simulink model "ModelPlant_DP_v3"  (R2015a)
settings: Solver=ode3  StartTime=0.0  StopTime=Simulation_Time  FixedStep=0.01  RelTol=1e-3
values from neighbouring files (symbols this model uses):
  DesiredPath = 0    [Innput.m]    (also in Input_v3.m = 1)
  Elipscenter_radi = [6 5;0 3 ]    [Innput.m]    (also in Input_v3.m)
  eta_dot_ini = [7;0;0]    [Innput.m]    (also in Input_v3.m)
  K = [2;10]    [Input_v3.m]
  K1 = diag([1,1,4])    [Input_v3.m]
  K2 = diag([200,50,3])    [Input_v3.m]    (also in inputDPgains.m = [1 0 0; 0 1 0; 0 0 1])
  l1 = [1 0 0;0 1 0;0 0 0.05]    [Input_v3.m]    (also in inputDPgains.m = [1 0 0; 0 1 0; 0 0 0.05])
  l2 = [1 0 0;0 1 0;0 0 0.05]    [Input_v3.m]    (also in inputDPgains.m = [1 0 0; 0 1 0; 0 0 0.05])
  l3 = [1 0 0;0 1 0;0 0 0.05]    [Input_v3.m]    (also in inputDPgains.m = [1 0 0; 0 1 0; 0 0 0.05])
  L_1 = 0.1    [Input_v3.m]
  L_2 = 2    [Input_v3.m]
  L_3 = 0.01    [Input_v3.m]
  LAW = 1    [Innput.m]    (also in Input_v3.m = 0)
  lim = [1.00;-20;6.45/2;-6.45/2]    [Innput.m]    (also in Input_v3.m = [20;-20;9;-9])
  lim_2 = [1.5;-22;7;-7]    [Innput.m]    (also in Input_v3.m = [25;-25;10;-10])
  m = 14.79    [Input_v3.m]    (also in ctrl_student_init.m)
  mu = mu(1)    [Innput.m]    (also in Input_v3.m = mu(2))
  pd = [2 10;0 4]    [Input_v3.m]
  T_initialDP = T_initialDP*100    (= 0)    [Input_v3.m]
  U_ref = 0.1    [Innput.m]    (also in Input_v3.m)
(part 1 of 2)
settings Model: CovSFcnEnable=off  Creator=Erik  LastModifiedBy=MCLab
settings DebuggingCC: SolverPrmCheckMsg=warning

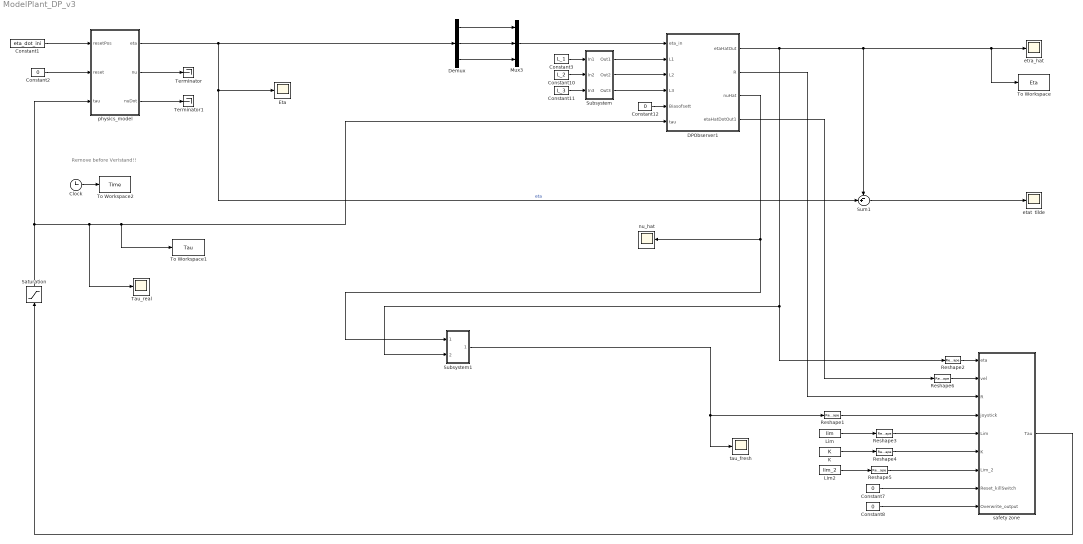
== system ModelPlant_DP_v3 ==
  note: Remove before Veristand!!
  Clock : Clock
  Constant1 : Constant  Value=eta_dot_ini
  Constant10 : Constant  Value=L_2
  Constant11 : Constant  Value=L_3
  Constant{2,7..8,12} (4 alike) : Constant  Value=0
  Constant3 : Constant  Value=L_1
  DPObserver1 : Subsystem
  Demux : Demux  Outputs=3
  Eta : Scope
      settings: TimeRange=1500  YMin=0  YMax=12  SaveName=ScopeData10
  K : Constant  Value=K
  Lim : Constant  Value=lim
  Lim2 : Constant  Value=lim_2
  Mux3 : Mux  Inputs=3
  Reshape1 : Reshape  OutputDimensionality=Customize  OutputDimensions=[3,1]
  Reshape2 : Reshape  OutputDimensionality=Customize  OutputDimensions=[3,1]
  Reshape3 : Reshape  OutputDimensionality=Customize  OutputDimensions=[4,1]
  Reshape4 : Reshape  OutputDimensionality=Customize  OutputDimensions=[2,1]
  Reshape5 : Reshape  OutputDimensionality=Customize  OutputDimensions=[4,1]
  Reshape6 : Reshape  OutputDimensionality=Customize  OutputDimensions=[3,1]
  Saturation : Saturate  UpperLimit=[1.03;2.5;0.98]  LowerLimit=-[1.03;2.5;0.98]
  Subsystem : Subsystem
  Subsystem1 : Subsystem
  Sum1 : Sum  Inputs=-+|
  Tau_real : Scope
      settings: YMin=-5e-05  YMax=0.0004  SaveName=ScopeData9
  Terminator : Terminator
  Terminator1 : Terminator
  To Workspace : ToWorkspace  VariableName=Eta  SampleTime=-1
  To Workspace1 : ToWorkspace  VariableName=Tau  SampleTime=-1
  To Workspace2 : ToWorkspace  VariableName=Time  SampleTime=-1
  etat  tilde : Scope
      settings: SaveName=ScopeData7
  etra_hat : Scope
      settings: YMin=0  YMax=25  SaveName=ScopeData5
  nu_hat : Scope
      settings: YMin=0  YMax=25  SaveName=ScopeData15
  physics_model : Subsystem
  "safety zone " : Subsystem
  tau_fresh : Scope
      settings: YMin=0  YMax=25  SaveName=ScopeData11
  wires:
  Demux/3 -> Mux3/3
  physics_model/1(eta) -> Sum1/2, Eta/1, Demux/1  "eta"
  Demux/1 -> Mux3/1
  Demux/2 -> Mux3/2
  Mux3/1 -> DPObserver1/1(eta_in)
  DPObserver1/3(nuHat) -> Subsystem1/1(nu_hat), nu_hat/1
  DPObserver1/4(etaHatDotOut1) -> Reshape6/1
  Subsystem/1(Out1) -> DPObserver1/2(L1)
  Subsystem/2(Out2) -> DPObserver1/3(L2)
  Subsystem/3(Out3) -> DPObserver1/4(L3)
  Constant7/1 -> "safety zone "/8(Reset_killSwitch)
  Constant8/1 -> "safety zone "/9(Overwrite_output)
  Lim/1 -> Reshape3/1
  K/1 -> Reshape4/1
  Lim2/1 -> Reshape5/1
  Reshape3/1 -> "safety zone "/5(Lim)
  Reshape4/1 -> "safety zone "/6(K)
  Reshape5/1 -> "safety zone "/7(Lim_2)
  Reshape1/1 -> "safety zone "/4(joystick)
  DPObserver1/2(R) -> "safety zone "/3(R)
  Reshape6/1 -> "safety zone "/2("vel ")
  Reshape2/1 -> "safety zone "/1(eta)
  Constant1/1 -> physics_model/1(resetPos)
  Constant2/1 -> physics_model/2(reset)
  physics_model/2(nu) -> Terminator/1
  physics_model/3(nuDot) -> Terminator1/1
  Constant3/1 -> Subsystem/1(In1)
  Constant11/1 -> Subsystem/3(In3)
  Constant10/1 -> Subsystem/2(In2)
  Constant12/1 -> DPObserver1/5(Biasofsett)
  "safety zone "/1(Tau) -> Saturation/1
  Saturation/1 -> physics_model/3(tau), Tau_real/1, To Workspace1/1, DPObserver1/6(tau)
  DPObserver1/1(etaHatOut) -> Reshape2/1, Subsystem1/2(Eta_hat), Sum1/1, To Workspace/1, etra_hat/1
  Sum1/1 -> etat  tilde/1
  Clock/1 -> To Workspace2/1
  Subsystem1/1(Tau) -> tau_fresh/1, Reshape1/1

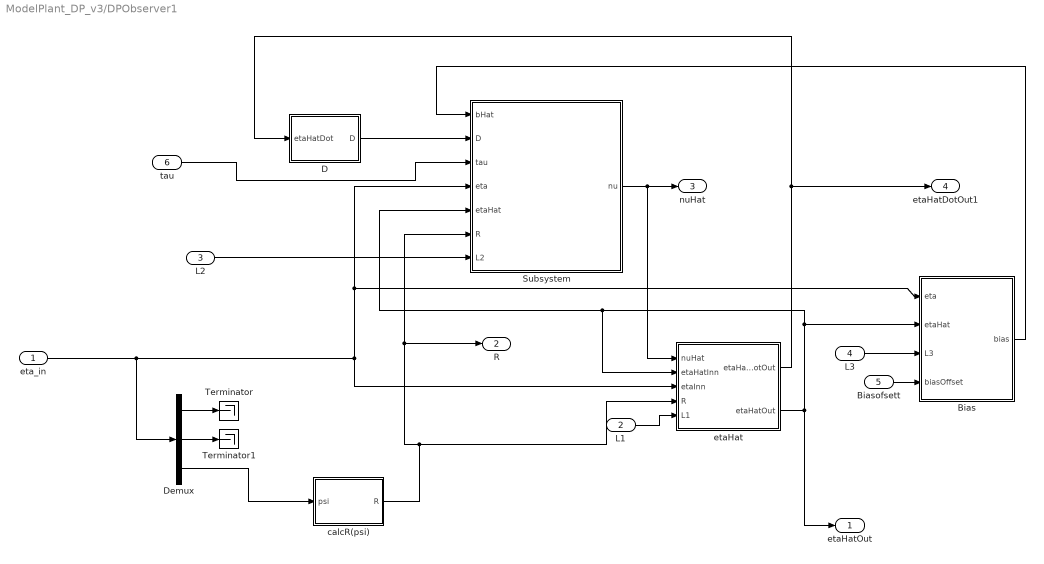
== system ModelPlant_DP_v3/DPObserver1 ==
  eta_in : Inport
  L1 : Inport  Port=2
  L2 : Inport  Port=3
  L3 : Inport  Port=4
  Biasofsett : Inport  Port=5
  tau : Inport  Port=6
  Bias : Subsystem
  D : MATLAB Function  TreatAsAtomicUnit=on
  Demux : Demux  Outputs=3
  Subsystem : Subsystem
  Terminator : Terminator
  Terminator1 : Terminator
  "calcR(psi) " : MATLAB Function  TreatAsAtomicUnit=on
  etaHat : Subsystem
  etaHatOut : Outport
  R : Outport  Port=2
  nuHat : Outport  Port=3
  etaHatDotOut1 : Outport  Port=4
  wires:
  "calcR(psi) "/1(R) -> R/1, Subsystem/6(R), etaHat/4(R)
  etaHat/2(etaHatOut) -> etaHatOut/1, Subsystem/5(etaHat), etaHat/2(etaHatInn), Bias/2(etaHat)
  tau/1 -> Subsystem/3(tau)
  etaHat/1(etaHatDotOut) -> etaHatDotOut1/1, D/1(etaHatDot)
  Subsystem/1(nu) -> nuHat/1, etaHat/1(nuHat)
  eta_in/1 -> Demux/1, etaHat/3(etaInn), Subsystem/4(eta), Bias/1(eta)
  D/1(D) -> Subsystem/2(D)
  Bias/1(bias) -> Subsystem/1(bHat)
  Demux/3 -> "calcR(psi) "/1(psi)
  L2/1 -> Subsystem/7(L2)
  L3/1 -> Bias/3(L3)
  Biasofsett/1 -> Bias/4(biasOffset)
  Demux/1 -> Terminator/1
  Demux/2 -> Terminator1/1
  L1/1 -> etaHat/5(L1)

== system ModelPlant_DP_v3/Subsystem ==
  In1 : Inport
  In2 : Inport  Port=2
  In3 : Inport  Port=3
  Constant1 : Constant  Value=l1
  Constant2 : Constant  Value=l2
  Constant3 : Constant  Value=l3
  Product : Product
  Product1 : Product
  Product2 : Product
  Out1 : Outport
  Out2 : Outport  Port=2
  Out3 : Outport  Port=3
  wires:
  Product/1 -> Out3/1
  Product2/1 -> Out2/1
  In3/1 -> Product/1
  Constant3/1 -> Product/2
  In2/1 -> Product2/1
  Constant2/1 -> Product2/2
  In1/1 -> Product1/1
  Constant1/1 -> Product1/2
  Product1/1 -> Out1/1

== system ModelPlant_DP_v3/Subsystem1 ==
  nu_hat : Inport
  Eta_hat : Inport  Port=2
  Controller1 : Subsystem
  Eta_dss : Scope
      settings: YMin=-2  YMax=10  SaveName=ScopeData14
  PathParameterization : Subsystem
  To Workspace3 : ToWorkspace  VariableName=pd_data  SampleTime=-1
  Tau : Outport
  wires:
  nu_hat/1 -> Controller1/1(nu_hat)
  Eta_hat/1 -> Controller1/8(eta_hat)
  Controller1/1("V_1s ") -> PathParameterization/1(V_1s)
  PathParameterization/3(s_dot) -> Controller1/4(s_dot)
  PathParameterization/2(U_s) -> Controller1/3(U_s)
  PathParameterization/1(eta_ds) -> Controller1/2("eta_ds ")
  PathParameterization/6(p_d_out) -> To Workspace3/1, Eta_dss/1, Controller1/7(p_d_in)
  PathParameterization/4(eta_dss) -> Controller1/5(eta_dss)
  PathParameterization/5(U_ss) -> Controller1/6(U_ss)
  Controller1/2(tau) -> Tau/1

== system ModelPlant_DP_v3/physics_model ==
  resetPos : Inport
  reset : Inport  Port=2
  tau : Inport  Port=3
  Integrator : Integrator  ExternalReset=rising  InitialCondition=[0 0 0]'
  Integrator1 : Integrator  ExternalReset=rising  InitialConditionSource=external  InitialCondition=[0 0 0]'
  Reshape1 : Reshape  OutputDimensionality=Customize  OutputDimensions=[3,1]
  Reshape3 : Reshape  OutputDimensionality=Customize  OutputDimensions=[3,1]
  kinematics : MATLAB Function  TreatAsAtomicUnit=on
  kinetics : MATLAB Function  TreatAsAtomicUnit=on
  eta : Outport
  nu : Outport  Port=2
  nuDot : Outport  Port=3
  wires:
  kinetics/1(nu_dot) -> nuDot/1, Integrator/1
  Integrator/1 -> nu/1, kinetics/2(nu), Reshape3/1
  kinematics/1(eta_dot) -> Integrator1/1
  reset/1 -> Integrator1/2, Integrator/2
  resetPos/1 -> Integrator1/3
  tau/1 -> kinetics/1(tau)
  Reshape3/1 -> kinematics/1(nu)
  Reshape1/1 -> kinematics/2(eta)
  Integrator1/1 -> Reshape1/1, eta/1

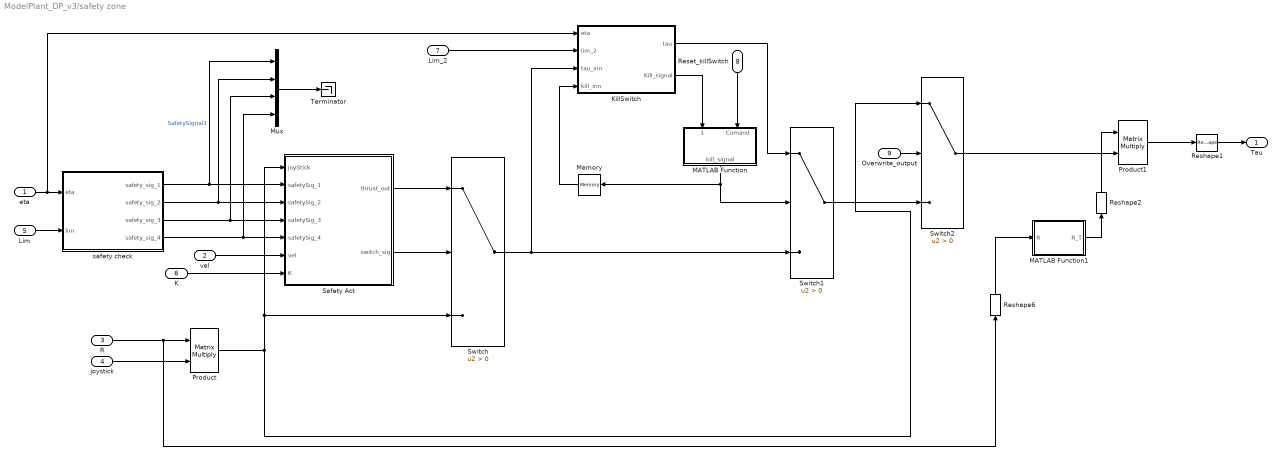
== system ModelPlant_DP_v3/safety zone  ==
  eta : Inport
  "vel " : Inport  Port=2
  R : Inport  Port=3
  joystick : Inport  Port=4
  Lim : Inport  Port=5
  K : Inport  Port=6
  Lim_2 : Inport  Port=7
  Reset_killSwitch : Inport  Port=8
  Overwrite_output : Inport  Port=9
  KillSwitch : MATLAB Function  TreatAsAtomicUnit=on
  MATLAB Function : MATLAB Function  TreatAsAtomicUnit=on
  MATLAB Function1 : MATLAB Function  TreatAsAtomicUnit=on
  Memory : Memory
  Mux : Mux
  Product : Product  Multiplication=Matrix(*)
  Product1 : Product  Multiplication=Matrix(*)
  Reshape1 : Reshape  OutputDimensionality=Customize  OutputDimensions=[3,1]
  Reshape2 : Reshape  OutputDimensionality=Customize  OutputDimensions=[3,3]
  Reshape6 : Reshape  OutputDimensionality=Customize  OutputDimensions=[3,3]
  Safety Act : MATLAB Function  TreatAsAtomicUnit=on
  Switch : Switch  Criteria=u2 > Threshold
  Switch1 : Switch  Criteria=u2 > Threshold
  Switch2 : Switch  Criteria=u2 > Threshold
  Terminator : Terminator
  safety check : MATLAB Function  TreatAsAtomicUnit=on
  Tau : Outport
  wires:
  safety check/1(safety_sig_1) -> Mux/1, Safety Act/2(safetySig_1)  "SafetySignal1"
  Safety Act/1(thrust_out) -> Switch/1
  safety check/2(safety_sig_2) -> Mux/2, Safety Act/3(safetySig_2)
  safety check/3(safety_sig_3) -> Safety Act/4(safetySig_3), Mux/3
  safety check/4(safety_sig_4) -> Safety Act/5(safetySig_4), Mux/4
  "vel "/1 -> Safety Act/6(vel)
  Mux/1 -> Terminator/1
  Lim/1 -> safety check/2(lim)
  Safety Act/2(switch_sig) -> Switch/2
  K/1 -> Safety Act/7(K)
  eta/1 -> KillSwitch/1(eta), safety check/1(eta)
  Lim_2/1 -> KillSwitch/2(lim_2)
  Memory/1 -> KillSwitch/4(kill_inn)
  Switch/1 -> KillSwitch/3(tau_inn), Switch1/3
  KillSwitch/1(tau) -> Switch1/1
  MATLAB Function/1(kill_signal) -> Memory/1, Switch1/2
  Reset_killSwitch/1 -> MATLAB Function/2(Comand)
  Overwrite_output/1 -> Switch2/2
  Switch1/1 -> Switch2/3
  KillSwitch/2(Kill_signal) -> MATLAB Function/1(kill_signalInn)
  R/1 -> Reshape6/1, Product/1
  joystick/1 -> Product/2
  Product/1 -> Safety Act/1(joyStick), Switch/3, Switch2/1
  MATLAB Function1/1(R_T) -> Reshape2/1
  Product1/1 -> Reshape1/1
  Reshape1/1 -> Tau/1
  Switch2/1 -> Product1/2
  Reshape6/1 -> MATLAB Function1/1(R)
  Reshape2/1 -> Product1/1

== system ModelPlant_DP_v3/DPObserver1/Bias ==
  eta : Inport
  etaHat : Inport  Port=2
  L3 : Inport  Port=3
  biasOffset : Inport  Port=4  PortDimensions=1
  Constant : Constant  Value=[1;1;1]
  IC1 : InitialCondition  Value=[0;0;0]
  Product : Product
  Sum : Sum  Inputs=|++
  bHat : Integrator
  bHatDot : MATLAB Function  TreatAsAtomicUnit=on
  bias : Outport
  wires:
  bHatDot/1(bHatDot) -> bHat/1
  eta/1 -> bHatDot/2(eta)
  etaHat/1 -> bHatDot/3(etaHat)
  L3/1 -> bHatDot/1(L3)
  IC1/1 -> bias/1
  Sum/1 -> IC1/1
  biasOffset/1 -> Product/1
  Product/1 -> Sum/2
  Constant/1 -> Product/2
  bHat/1 -> Sum/1

== system ModelPlant_DP_v3/DPObserver1/Subsystem ==
  bHat : Inport
  D : Inport  Port=2
  tau : Inport  Port=3
  eta : Inport  Port=4
  etaHat : Inport  Port=5
  R : Inport  Port=6
  L2 : Inport  Port=7
  IC : InitialCondition  Value=[0;0;0]
  M : MATLAB Function  TreatAsAtomicUnit=on
  nuHat : Integrator  InitialCondition=[0;0;0]
  nuHatDot : MATLAB Function  TreatAsAtomicUnit=on
  nu : Outport
  wires:
  tau/1 -> nuHatDot/6(tau)
  bHat/1 -> nuHatDot/2(bHat)
  M/1(M) -> nuHatDot/4(M)
  nuHat/1 -> nuHatDot/1(nuHat), nu/1
  etaHat/1 -> nuHatDot/9(etaHat)
  R/1 -> nuHatDot/8(R)
  eta/1 -> nuHatDot/7(eta)
  nuHatDot/1(nuHatDot) -> IC/1
  D/1 -> nuHatDot/3(D)
  L2/1 -> nuHatDot/5(L2)
  IC/1 -> nuHat/1

== system ModelPlant_DP_v3/DPObserver1/etaHat ==
  nuHat : Inport
  etaHatInn : Inport  Port=2
  etaInn : Inport  Port=3
  R : Inport  Port=4
  L1 : Inport  Port=5
  etaHat : Integrator  InitialCondition=eta_dot_ini
  etaHatDot : MATLAB Function  TreatAsAtomicUnit=on
  etaHatDotOut : Outport
  etaHatOut : Outport  Port=2
  wires:
  etaHat/1 -> etaHatOut/1
  etaHatDot/1(etaHatDot) -> etaHat/1, etaHatDotOut/1
  L1/1 -> etaHatDot/3(L1)
  R/1 -> etaHatDot/5(R)
  nuHat/1 -> etaHatDot/2(nuHat)
  etaInn/1 -> etaHatDot/4(eta)
  etaHatInn/1 -> etaHatDot/1(etaHat)

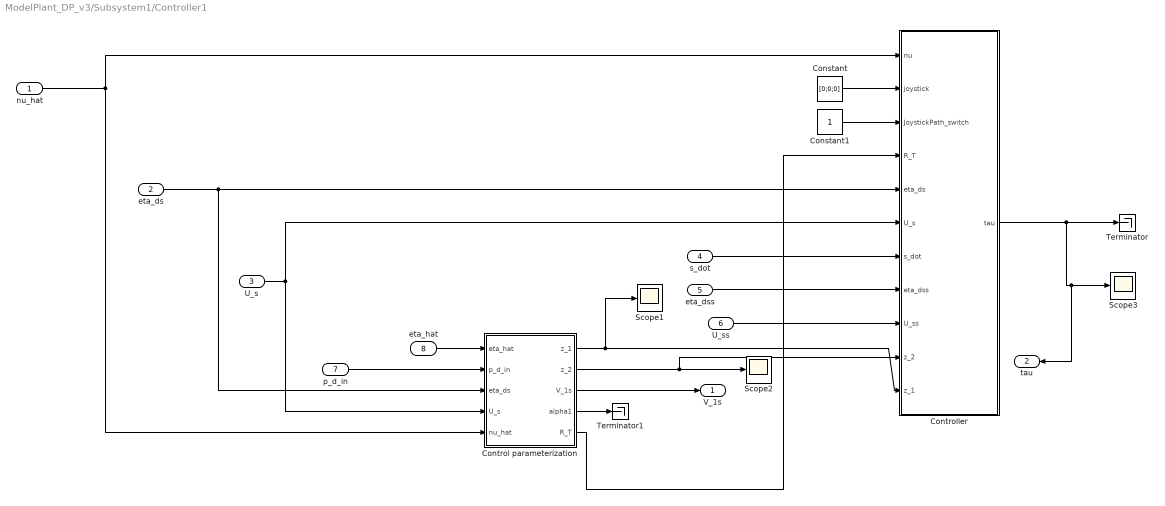
== system ModelPlant_DP_v3/Subsystem1/Controller1 ==
  nu_hat : Inport
  "eta_ds " : Inport  Port=2
  U_s : Inport  Port=3
  s_dot : Inport  Port=4
  eta_dss : Inport  Port=5
  U_ss : Inport  Port=6
  p_d_in : Inport  Port=7
  eta_hat : Inport  Port=8
  Constant : Constant  Value=[0;0;0]
  Constant1 : Constant
  Control parameterization : Subsystem
  Controller : Subsystem
  Scope1 : Scope
      settings: YMin=-6.76763  YMax=7.09799  SaveName=ScopeData8
  Scope2 : Scope
  Scope3 : Scope
      settings: YMin=-11.79233  YMax=2.58486  SaveName=ScopeData3
  Terminator : Terminator
  Terminator1 : Terminator
  "V_1s " : Outport
  tau : Outport  Port=2
  wires:
  Control parameterization/1(z_1) -> Scope1/1, Controller/11(z_1)
  Control parameterization/2(z_2) -> Scope2/1, Controller/10(z_2)
  nu_hat/1 -> Controller/1(" nu"), Control parameterization/5(nu_hat)
  Control parameterization/5("R_T ") -> Controller/4(R_T)
  Constant/1 -> Controller/2(joystick)
  Constant1/1 -> Controller/3(JoystickPath_switch)
  Controller/1(tau) -> tau/1, Scope3/1, Terminator/1
  Control parameterization/4(alpha1) -> Terminator1/1
  U_ss/1 -> Controller/9(U_ss)
  s_dot/1 -> Controller/7(s_dot)
  eta_dss/1 -> Controller/8(eta_dss)
  Control parameterization/3("V_1s ") -> "V_1s "/1
  U_s/1 -> Controller/6(U_s), Control parameterization/4(U_s)
  "eta_ds "/1 -> Control parameterization/3("eta_ds "), Controller/5(eta_ds)
  p_d_in/1 -> Control parameterization/2("p_d_in ")
  eta_hat/1 -> Control parameterization/1(eta_hat)

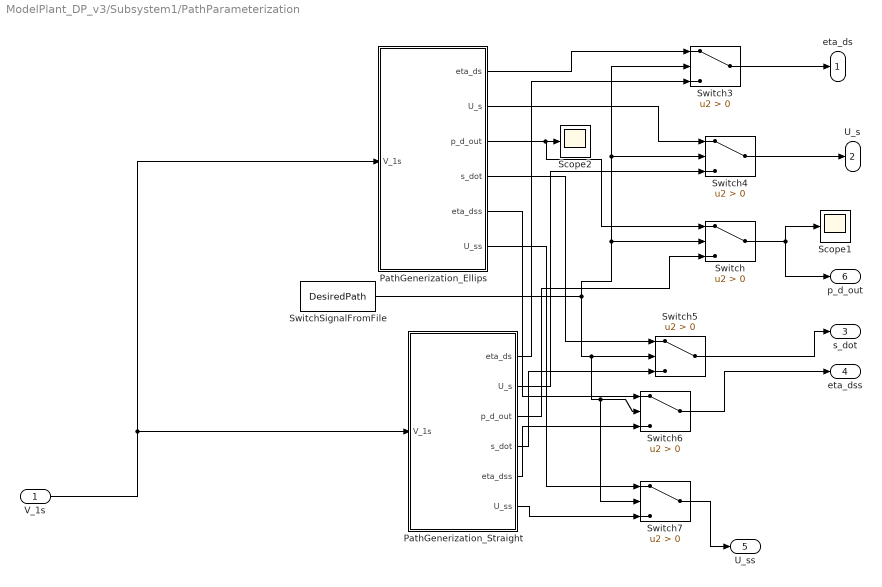
== system ModelPlant_DP_v3/Subsystem1/PathParameterization ==
  V_1s : Inport
  PathGenerization_Ellips : Subsystem
  PathGenerization_Straight : Subsystem
  Scope1 : Scope
      settings: YMin=-1.25  YMax=11.25  SaveName=ScopeData2
  Scope2 : Scope
      settings: YMin=-4.75  YMax=12.75  SaveName=ScopeData12
  Switch{,3..7} (6 alike) : Switch  Criteria=u2 > Threshold
  SwitchSignalFromFile : Constant  Value=DesiredPath
  eta_ds : Outport
  U_s : Outport  Port=2
  s_dot : Outport  Port=3
  eta_dss : Outport  Port=4
  U_ss : Outport  Port=5
  p_d_out : Outport  Port=6
  wires:
  PathGenerization_Ellips/4(s_dot) -> Switch5/1
  PathGenerization_Straight/4(s_dot) -> Switch5/3
  PathGenerization_Ellips/6(U_ss) -> Switch7/1
  PathGenerization_Straight/6(U_ss) -> Switch7/3
  PathGenerization_Straight/5("eta_dss ") -> Switch6/3
  PathGenerization_Straight/1(eta_ds) -> Switch3/3
  PathGenerization_Ellips/1(eta_ds) -> Switch3/1
  PathGenerization_Straight/2(U_s) -> Switch4/3
  PathGenerization_Straight/3(p_d_out) -> Switch/3
  PathGenerization_Ellips/2(U_s) -> Switch4/1
  PathGenerization_Ellips/3(p_d_out) -> Switch/1, Scope2/1
  SwitchSignalFromFile/1 -> Switch4/2, Switch3/2, Switch/2, Switch7/2, Switch6/2, Switch5/2
  Switch3/1 -> eta_ds/1
  Switch4/1 -> U_s/1
  Switch5/1 -> s_dot/1
  Switch6/1 -> eta_dss/1
  Switch7/1 -> U_ss/1
  V_1s/1 -> PathGenerization_Ellips/1(V_1s), PathGenerization_Straight/1(V_1s)
  Switch/1 -> p_d_out/1, Scope1/1
  PathGenerization_Ellips/5("eta_dss ") -> Switch6/1

== system ModelPlant_DP_v3/Subsystem1/Controller1/Control parameterization ==
  eta_hat : Inport
  "p_d_in " : Inport  Port=2
  "eta_ds " : Inport  Port=3
  U_s : Inport  Port=4
  nu_hat : Inport  Port=5
  "BacksteppingParameterization " : Subsystem
  z_1 : Outport
  z_2 : Outport  Port=2
  "V_1s " : Outport  Port=3
  alpha1 : Outport  Port=4
  "R_T " : Outport  Port=5
  wires:
  "eta_ds "/1 -> "BacksteppingParameterization "/3(eta_ds)
  eta_hat/1 -> "BacksteppingParameterization "/1(eta_hat)
  "p_d_in "/1 -> "BacksteppingParameterization "/2("p_d_in ")
  "BacksteppingParameterization "/1(V_1s_out) -> "V_1s "/1
  U_s/1 -> "BacksteppingParameterization "/4(U_s)
  "BacksteppingParameterization "/3(z_2) -> z_2/1
  nu_hat/1 -> "BacksteppingParameterization "/5(nu_hat)
  "BacksteppingParameterization "/2(z_1) -> z_1/1
  "BacksteppingParameterization "/4("alpha1 ") -> alpha1/1
  "BacksteppingParameterization "/5(R_T) -> "R_T "/1

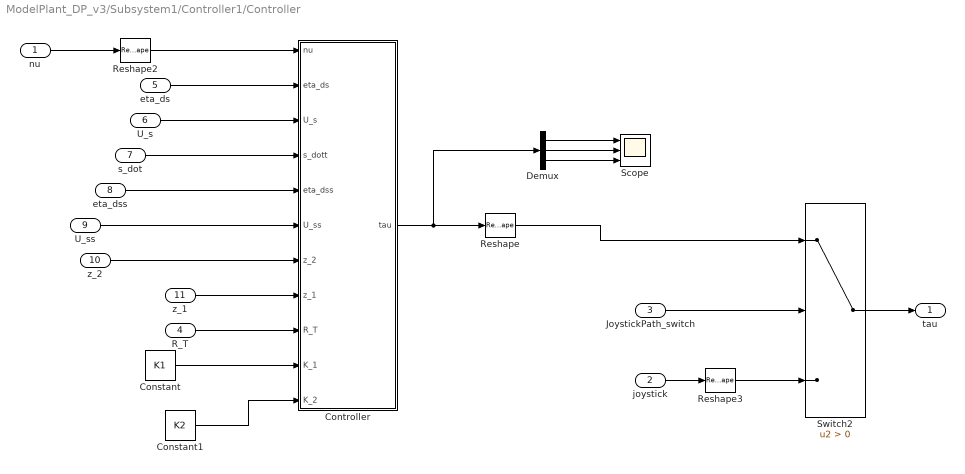
== system ModelPlant_DP_v3/Subsystem1/Controller1/Controller ==
  " nu" : Inport
  joystick : Inport  Port=2
  JoystickPath_switch : Inport  Port=3
  R_T : Inport  Port=4
  eta_ds : Inport  Port=5
  U_s : Inport  Port=6
  s_dot : Inport  Port=7
  eta_dss : Inport  Port=8
  U_ss : Inport  Port=9
  z_2 : Inport  Port=10
  z_1 : Inport  Port=11
  Constant : Constant  Value=K1
  Constant1 : Constant  Value=K2
  Controller : Subsystem
  Demux : Demux  Outputs=3
  Reshape : Reshape  OutputDimensionality=Customize  OutputDimensions=[3,1]
  Reshape2 : Reshape  OutputDimensionality=Customize  OutputDimensions=[3,1]
  Reshape3 : Reshape  OutputDimensionality=Customize  OutputDimensions=[3,1]
  Scope : Scope  NumInputPorts=3
      settings: YMin=-1.81121~-0.05182~-0.00671  YMax=5.53458~0.46636~0.06037  SaveName=ScopeData6
  Switch2 : Switch  Criteria=u2 > Threshold
  tau : Outport
  wires:
  " nu"/1 -> Reshape2/1
  Switch2/1 -> tau/1
  joystick/1 -> Reshape3/1
  JoystickPath_switch/1 -> Switch2/2
  eta_ds/1 -> Controller/2(eta_ds)
  U_s/1 -> Controller/3(U_s)
  s_dot/1 -> Controller/4(s_dott)
  eta_dss/1 -> Controller/5(eta_dss)
  U_ss/1 -> Controller/6(U_ss)
  Controller/1(tau) -> Demux/1, Reshape/1
  R_T/1 -> Controller/9(R_T)
  Constant/1 -> Controller/10(K_1)
  Constant1/1 -> Controller/11(K_2)
  Reshape/1 -> Switch2/1
  z_2/1 -> Controller/7(z_2)
  Reshape2/1 -> Controller/1(nu)
  Reshape3/1 -> Switch2/3
  z_1/1 -> Controller/8(z_1)
  Demux/1 -> Scope/1
  Demux/2 -> Scope/2
  Demux/3 -> Scope/3

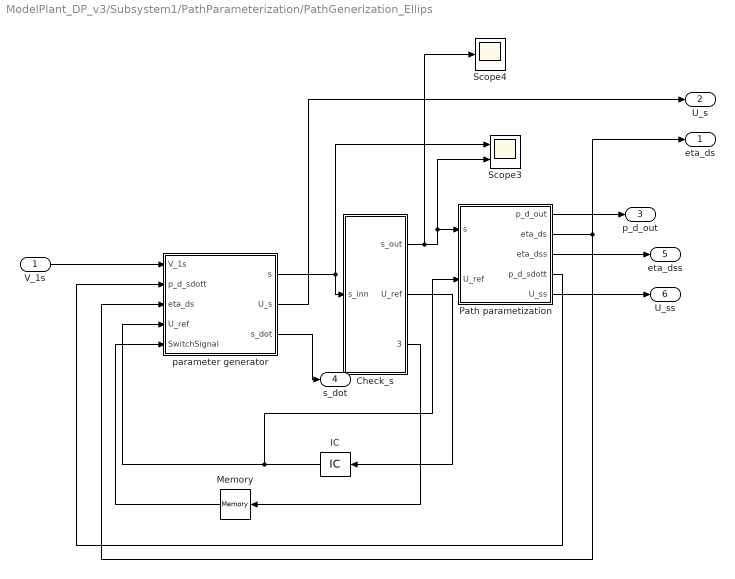
== system ModelPlant_DP_v3/Subsystem1/PathParameterization/PathGenerization_Ellips ==
  V_1s : Inport
  Check_s : Subsystem
  IC : InitialCondition  Value=0
  Memory : Memory
  "Path parametization " : Subsystem
  Scope3 : Scope  NumInputPorts=2
      settings: YMin=-0.125  YMax=1.12502  SaveName=ScopeData13
  Scope4 : Scope
  parameter generator : Subsystem
  eta_ds : Outport
  U_s : Outport  Port=2
  p_d_out : Outport  Port=3
  s_dot : Outport  Port=4
  "eta_dss " : Outport  Port=5
  U_ss : Outport  Port=6
  wires:
  "Path parametization "/1("p_d_out ") -> p_d_out/1
  parameter generator/1(s) -> Scope3/1, Check_s/1(s_inn)
  "Path parametization "/4(p_d_sdott) -> parameter generator/2(p_d_sdott)
  parameter generator/2(U_s) -> U_s/1
  "Path parametization "/2("eta_ds ") -> parameter generator/3(eta_ds), eta_ds/1
  V_1s/1 -> parameter generator/1(V_1s)
  Check_s/1(s_out) -> Scope4/1, Scope3/2, "Path parametization "/1(s)
  Check_s/2(U_ref) -> IC/1
  IC/1 -> "Path parametization "/2(U_ref), parameter generator/4(U_ref)
  Memory/1 -> parameter generator/5(SwitchSignal)
  Check_s/3(SwitchSignal) -> Memory/1
  parameter generator/3("s_dot ") -> s_dot/1
  "Path parametization "/3(eta_dss) -> "eta_dss "/1
  "Path parametization "/5(U_ss) -> U_ss/1

== system ModelPlant_DP_v3/Subsystem1/PathParameterization/PathGenerization_Straight ==
  V_1s : Inport
  IC : InitialCondition  Value=0
  Memory : Memory
  "Path parametization " : Subsystem
  Scope1 : Scope
  Scope3 : Scope
  parameter generator : Subsystem
  eta_ds : Outport
  U_s : Outport  Port=2
  p_d_out : Outport  Port=3
  s_dot : Outport  Port=4
  "eta_dss " : Outport  Port=5
  U_ss : Outport  Port=6
  wires:
  "Path parametization "/1("p_d_out ") -> p_d_out/1
  "Path parametization "/3(p_d_sdott) -> parameter generator/2(p_d_sdott)
  "Path parametization "/2("eta_ds ") -> parameter generator/3(eta_ds), eta_ds/1
  V_1s/1 -> parameter generator/1(V_1s)
  parameter generator/1(s) -> Scope3/1, "Path parametization "/1(s)
  IC/1 -> parameter generator/4(U_ref)
  Memory/1 -> parameter generator/5(SwitchSignal)
  "Path parametization "/4(SwitchSignal) -> Memory/1
  parameter generator/3("s_dot ") -> s_dot/1
  "Path parametization "/5(eta_dss) -> "eta_dss "/1
  "Path parametization "/6(U_ss) -> U_ss/1
  parameter generator/2(U_s) -> Scope1/1, U_s/1
  "Path parametization "/7(U) -> IC/1

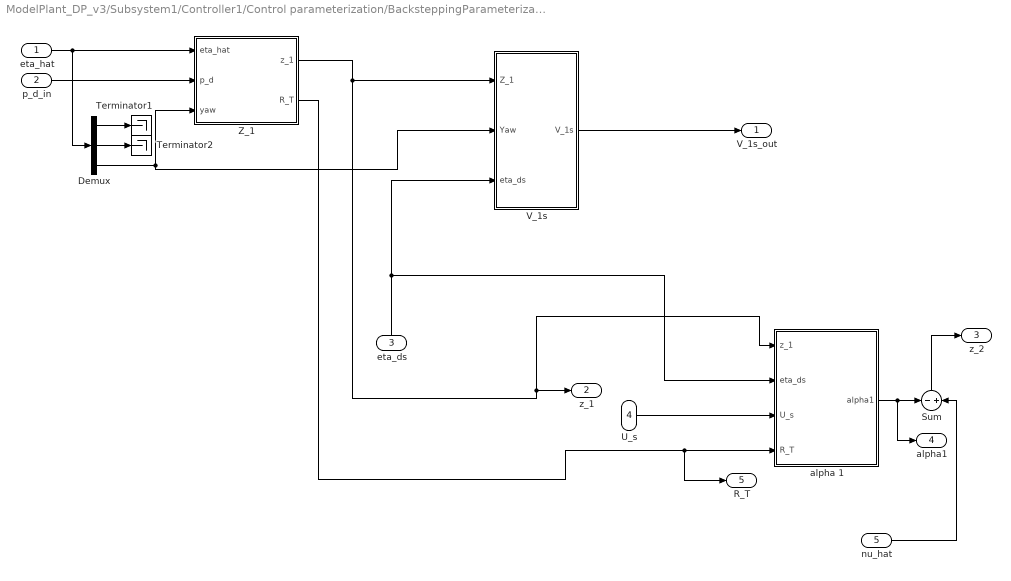
== system ModelPlant_DP_v3/Subsystem1/Controller1/Control parameterization/BacksteppingParameterization  ==
  eta_hat : Inport
  "p_d_in " : Inport  Port=2
  eta_ds : Inport  Port=3
  U_s : Inport  Port=4
  nu_hat : Inport  Port=5
  Demux : Demux  Outputs=3
  Sum : Sum  Inputs=-|+
  Terminator1 : Terminator
  Terminator2 : Terminator
  V_1s : Subsystem
  Z_1 : Subsystem
  alpha 1 : Subsystem
  V_1s_out : Outport
  z_1 : Outport  Port=2
  z_2 : Outport  Port=3
  "alpha1 " : Outport  Port=4
  R_T : Outport  Port=5
  wires:
  eta_ds/1 -> alpha 1/2(eta_ds), V_1s/3(eta_ds)
  eta_hat/1 -> Demux/1, Z_1/1(eta_hat)
  "p_d_in "/1 -> Z_1/2(p_d)
  Demux/3 -> V_1s/2(Yaw), Z_1/3("yaw ")
  V_1s/1(V_1s) -> V_1s_out/1
  alpha 1/1(alpha1) -> "alpha1 "/1, Sum/1
  U_s/1 -> alpha 1/3(U_s)
  Z_1/1(z_1) -> alpha 1/1(z_1), z_1/1, V_1s/1(Z_1)
  Z_1/2(R_T) -> R_T/1, alpha 1/4(R_T)
  nu_hat/1 -> Sum/2
  Sum/1 -> z_2/1
  Demux/1 -> Terminator1/1
  Demux/2 -> Terminator2/1

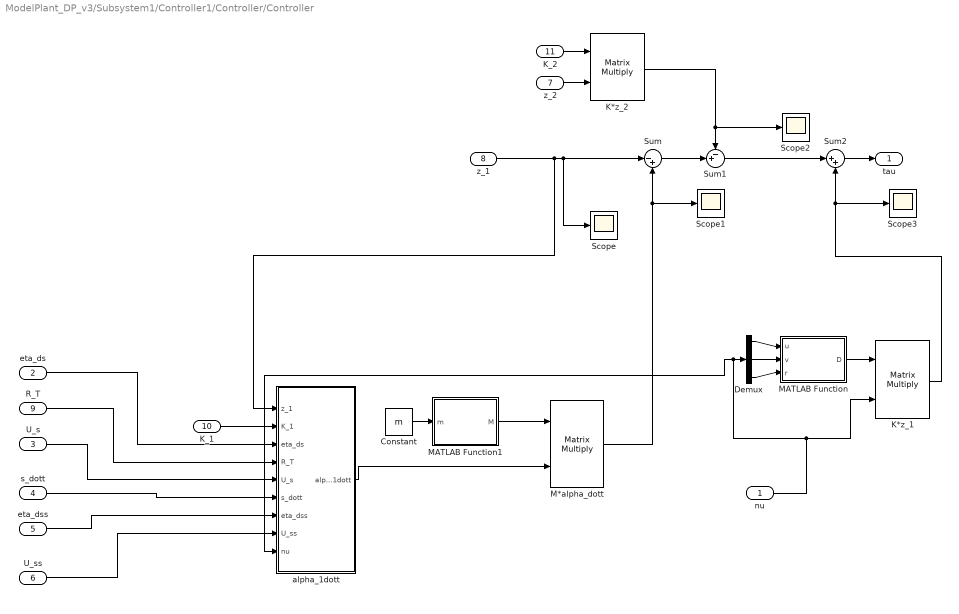
== system ModelPlant_DP_v3/Subsystem1/Controller1/Controller/Controller ==
  nu : Inport
  eta_ds : Inport  Port=2
  U_s : Inport  Port=3
  s_dott : Inport  Port=4
  eta_dss : Inport  Port=5
  U_ss : Inport  Port=6
  z_2 : Inport  Port=7
  z_1 : Inport  Port=8
  R_T : Inport  Port=9
  K_1 : Inport  Port=10
  K_2 : Inport  Port=11
  Constant : Constant  Value=m
  Demux : Demux  Outputs=3
  K*z_1 : Product  Multiplication=Matrix(*)
  K*z_2 : Product  Multiplication=Matrix(*)
  M*alpha_dott : Product  Multiplication=Matrix(*)
  MATLAB Function : MATLAB Function  TreatAsAtomicUnit=on
  MATLAB Function1 : MATLAB Function  TreatAsAtomicUnit=on
  Scope{,1..3} (4 alike) : Scope
      Scope settings: YMin=-1.86769  YMax=9.78914
      Scope1 settings: YMin=-0.31241  YMax=0.96684  SaveName=ScopeData2
      Scope2 settings: YMin=-1.22848  YMax=2.91428  SaveName=ScopeData3
      Scope3 settings: YMin=-1.62155  YMax=0.35636  SaveName=ScopeData4
  Sum : Sum  Inputs=|-+
  Sum1 : Sum  Inputs=-+|
  Sum2 : Sum  Inputs=|++
  alpha_1dott : Subsystem
  tau : Outport
  wires:
  alpha_1dott/1(alpha_1dott) -> M*alpha_dott/2
  MATLAB Function1/1(M) -> M*alpha_dott/1
  z_1/1 -> alpha_1dott/1(z_1), Scope/1, Sum/1
  Sum/1 -> Sum1/2
  Sum1/1 -> Sum2/1
  Sum2/1 -> tau/1
  z_2/1 -> K*z_2/2
  K*z_1/1 -> Sum2/2, Scope3/1
  nu/1 -> alpha_1dott/9(nu), Demux/1, K*z_1/2
  eta_ds/1 -> alpha_1dott/3(eta_ds)
  R_T/1 -> alpha_1dott/4(R_T)
  U_s/1 -> alpha_1dott/5(U_s)
  s_dott/1 -> alpha_1dott/6(s_dott)
  eta_dss/1 -> alpha_1dott/7(eta_dss)
  U_ss/1 -> alpha_1dott/8(U_ss)
  K_1/1 -> alpha_1dott/2(K_1)
  K_2/1 -> K*z_2/1
  Demux/1 -> MATLAB Function/1(u)
  Demux/2 -> MATLAB Function/2(v)
  Demux/3 -> MATLAB Function/3(r)
  MATLAB Function/1(D) -> K*z_1/1
  Constant/1 -> MATLAB Function1/1(m)
  K*z_2/1 -> Scope2/1, Sum1/1
  M*alpha_dott/1 -> Scope1/1, Sum/2

== system ModelPlant_DP_v3/Subsystem1/PathParameterization/PathGenerization_Ellips/Check_s ==
  s_inn : Inport
  CheckS&getU : MATLAB Function  TreatAsAtomicUnit=on
  Constant : Constant  Value=U_ref
  s_out : Outport
  U_ref : Outport  Port=2
  SwitchSignal : Outport  Port=3
  wires:
  CheckS&getU/1(s_out) -> s_out/1
  s_inn/1 -> CheckS&getU/1(s_inn)
  CheckS&getU/2(U) -> U_ref/1
  Constant/1 -> CheckS&getU/2(U_ref)
  CheckS&getU/3(Switch) -> SwitchSignal/1

== system ModelPlant_DP_v3/Subsystem1/PathParameterization/PathGenerization_Ellips/Path parametization  ==
  s : Inport
  U_ref : Inport  Port=2
  Elipscenter_radi : Constant  Value=Elipscenter_radi  VectorParams1D=off
  Subsystem : Subsystem
  "p_d_out " : Outport
  "eta_ds " : Outport  Port=2
  eta_dss : Outport  Port=3
  p_d_sdott : Outport  Port=4
  U_ss : Outport  Port=5
  wires:
  Elipscenter_radi/1 -> Subsystem/1(Elipscenter_radi)
  s/1 -> Subsystem/2(s)
  Subsystem/1(P_d) -> "p_d_out "/1
  Subsystem/2(Pd_s) -> p_d_sdott/1
  Subsystem/3(eta_ds) -> "eta_ds "/1
  Subsystem/4(eta_dss) -> eta_dss/1
  U_ref/1 -> Subsystem/3(U_ref)
  Subsystem/5(U_ss) -> U_ss/1

== system ModelPlant_DP_v3/Subsystem1/PathParameterization/PathGenerization_Ellips/parameter generator ==
  V_1s : Inport
  p_d_sdott : Inport  Port=2
  eta_ds : Inport  Port=3
  U_ref : Inport  Port=4
  SwitchSignal : Inport  Port=5
  Integrator : Integrator  ExternalReset=rising
  MATLAB Function1 : MATLAB Function  TreatAsAtomicUnit=on
  TASK : Constant  Value=LAW
  UpdateLaw : MATLAB Function  TreatAsAtomicUnit=on
  "mu " : Constant  Value=mu
  s : Outport
  U_s : Outport  Port=2
  "s_dot " : Outport  Port=3
  wires:
  Integrator/1 -> s/1
  p_d_sdott/1 -> UpdateLaw/1(p_d_sdot)
  UpdateLaw/1(s_dot) -> "s_dot "/1, Integrator/1
  UpdateLaw/2(U_s) -> U_s/1
  U_ref/1 -> UpdateLaw/2(U_ref)
  V_1s/1 -> UpdateLaw/3(V_1s)
  "mu "/1 -> UpdateLaw/4(mu)
  eta_ds/1 -> UpdateLaw/5(eta_ds)
  MATLAB Function1/1(SwitchSignal_Out) -> Integrator/2
  TASK/1 -> UpdateLaw/6(LAW)
  SwitchSignal/1 -> MATLAB Function1/1(SwitchSignal_In)

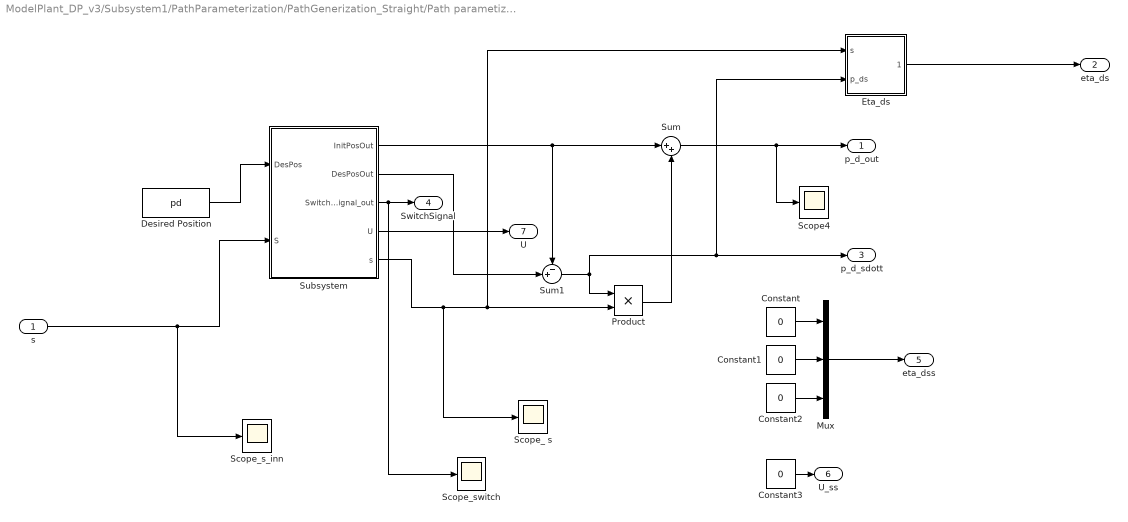
== system ModelPlant_DP_v3/Subsystem1/PathParameterization/PathGenerization_Straight/Path parametization  ==
  s : Inport
  Constant{,1..3} (4 alike) : Constant  Value=0
  Desired Position : Constant  Value=pd  VectorParams1D=off
  Eta_ds : Subsystem
  Mux : Mux  Inputs=3
  Product : Product
  Scope4 : Scope
      settings: YMin=0  YMax=12
  Scope_ s : Scope
      settings: YMin=0  YMax=1
  Scope_s_inn : Scope
      settings: TimeRange=1000  YMin=0  YMax=1.4
  Scope_switch : Scope
      settings: YMin=-0  YMax=2
  Subsystem : Subsystem
  Sum : Sum  Inputs=|++
  Sum1 : Sum  Inputs=-+|
  "p_d_out " : Outport
  "eta_ds " : Outport  Port=2
  p_d_sdott : Outport  Port=3
  SwitchSignal : Outport  Port=4
  eta_dss : Outport  Port=5
  U_ss : Outport  Port=6
  U : Outport  Port=7
  wires:
  Product/1 -> Sum/2
  Desired Position/1 -> Subsystem/1(DesPos)
  s/1 -> Scope_s_inn/1, Subsystem/2(S)
  Sum1/1 -> Product/1, Eta_ds/2(p_ds), p_d_sdott/1
  Eta_ds/1(eta_ds) -> "eta_ds "/1
  Subsystem/1(InitPosOut) -> Sum1/1, Sum/1
  Subsystem/3(SwitchSignal_out) -> Scope_switch/1, SwitchSignal/1
  Subsystem/2(DesPosOut) -> Sum1/2
  Sum/1 -> Scope4/1, "p_d_out "/1
  Mux/1 -> eta_dss/1
  Constant/1 -> Mux/1
  Constant1/1 -> Mux/2
  Constant2/1 -> Mux/3
  Constant3/1 -> U_ss/1
  Subsystem/4(U) -> U/1
  Subsystem/5(s) -> Scope_ s/1, Eta_ds/1(s), Product/2

== system ModelPlant_DP_v3/Subsystem1/PathParameterization/PathGenerization_Straight/parameter generator ==
  V_1s : Inport
  p_d_sdott : Inport  Port=2
  eta_ds : Inport  Port=3
  U_ref : Inport  Port=4
  SwitchSignal : Inport  Port=5
  Integrator : Integrator  ExternalReset=rising
  MATLAB Function1 : MATLAB Function  TreatAsAtomicUnit=on
  TASK : Constant  Value=LAW
  UpdateLaw : MATLAB Function  TreatAsAtomicUnit=on
  "mu " : Constant  Value=mu
  s : Outport
  U_s : Outport  Port=2
  "s_dot " : Outport  Port=3
  wires:
  Integrator/1 -> s/1
  p_d_sdott/1 -> UpdateLaw/1(p_d_sdot)
  UpdateLaw/1(s_dot) -> "s_dot "/1, Integrator/1
  UpdateLaw/2(U_s) -> U_s/1
  U_ref/1 -> UpdateLaw/2(U_ref)
  V_1s/1 -> UpdateLaw/3(V_1s)
  "mu "/1 -> UpdateLaw/4(mu)
  eta_ds/1 -> UpdateLaw/5(eta_ds)
  MATLAB Function1/1(SwitchSignal_Out) -> Integrator/2
  TASK/1 -> UpdateLaw/6(LAW)
  SwitchSignal/1 -> MATLAB Function1/1(SwitchSignal_In)

== system ModelPlant_DP_v3/Subsystem1/Controller1/Control parameterization/BacksteppingParameterization /V_1s ==
  Z_1 : Inport
  Yaw : Inport  Port=2
  eta_ds : Inport  Port=3
  Gain : Gain  Gain=-1
  MATLAB Function : MATLAB Function  TreatAsAtomicUnit=on
  MATLAB Function1 : MATLAB Function  TreatAsAtomicUnit=on
  Product : Product  Multiplication=Matrix(*)
  Product1 : Product  Multiplication=Matrix(*)
  Rotation Matrix : MATLAB Function  TreatAsAtomicUnit=on
  V_1s : Outport
  wires:
  Z_1/1 -> MATLAB Function/1(z_1)
  Rotation Matrix/1(R) -> MATLAB Function1/1(R)
  MATLAB Function1/1(R_T) -> Product/2
  Yaw/1 -> Rotation Matrix/1(yaw)
  MATLAB Function/1(z_1T) -> Product/1
  Product/1 -> Product1/1
  Product1/1 -> Gain/1
  eta_ds/1 -> Product1/2
  Gain/1 -> V_1s/1

== system ModelPlant_DP_v3/Subsystem1/Controller1/Control parameterization/BacksteppingParameterization /Z_1 ==
  eta_hat : Inport
  p_d : Inport  Port=2
  "yaw " : Inport  Port=3
  Mux : Mux  Inputs=2
  Product : Product  Multiplication=Matrix(*)
  R Transposed : MATLAB Function  TreatAsAtomicUnit=on
  Reshape1 : Reshape  OutputDimensionality=Customize  OutputDimensions=[3,3]
  Rotation Matrix : MATLAB Function  TreatAsAtomicUnit=on
  Sum : Sum  Inputs=|+-
  z_1 : Outport
  R_T : Outport  Port=2
  wires:
  "yaw "/1 -> Mux/2, Rotation Matrix/1(yaw)
  p_d/1 -> Mux/1
  Sum/1 -> Product/2
  Rotation Matrix/1(R) -> R Transposed/1(R)
  Product/1 -> z_1/1
  Mux/1 -> Sum/2
  R Transposed/1(R_T) -> Reshape1/1
  Reshape1/1 -> Product/1, R_T/1
  eta_hat/1 -> Sum/1

== system ModelPlant_DP_v3/Subsystem1/Controller1/Control parameterization/BacksteppingParameterization /alpha 1 ==
  z_1 : Inport
  eta_ds : Inport  Port=2
  U_s : Inport  Port=3
  R_T : Inport  Port=4
  Gain : Gain  Gain=-1
  "Kp " : Constant  Value=K1
  Product : Product  Multiplication=Matrix(*)
  Product1 : Product  Multiplication=Matrix(*)
  Product2 : Product  Multiplication=Matrix(*)
  Reshape : Reshape  OutputDimensionality=Customize  OutputDimensions=[3,1]
  Reshape1 : Reshape  OutputDimensionality=Customize
  Sum : Sum  Inputs=|++
  alpha1 : Outport
  wires:
  "Kp "/1 -> Gain/1
  Gain/1 -> Product/1
  z_1/1 -> Product/2
  Sum/1 -> alpha1/1
  Product/1 -> Sum/1
  Product1/1 -> Product2/2
  eta_ds/1 -> Reshape/1
  U_s/1 -> Reshape1/1
  Reshape/1 -> Product1/1
  Reshape1/1 -> Product1/2
  Product2/1 -> Sum/2
  R_T/1 -> Product2/1

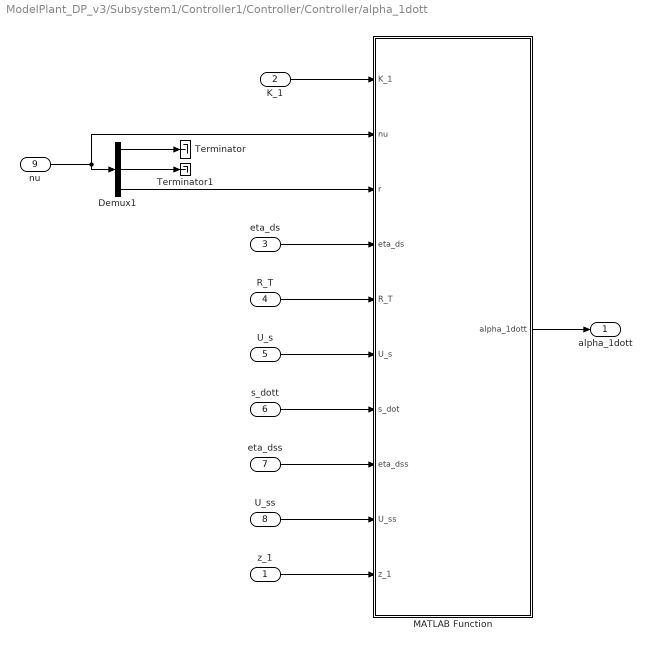
== system ModelPlant_DP_v3/Subsystem1/Controller1/Controller/Controller/alpha_1dott ==
  z_1 : Inport
  K_1 : Inport  Port=2
  eta_ds : Inport  Port=3
  R_T : Inport  Port=4
  U_s : Inport  Port=5
  s_dott : Inport  Port=6
  eta_dss : Inport  Port=7
  U_ss : Inport  Port=8
  nu : Inport  Port=9
  Demux1 : Demux  Outputs=3
  MATLAB Function : MATLAB Function  TreatAsAtomicUnit=on
  Terminator : Terminator
  Terminator1 : Terminator
  alpha_1dott : Outport
  wires:
  Demux1/1 -> Terminator/1
  Demux1/2 -> Terminator1/1
  nu/1 -> MATLAB Function/2(nu), Demux1/1
  Demux1/3 -> MATLAB Function/3(r)
  K_1/1 -> MATLAB Function/1(K_1)
  eta_ds/1 -> MATLAB Function/4(eta_ds)
  R_T/1 -> MATLAB Function/5(R_T)
  U_s/1 -> MATLAB Function/6(U_s)
  s_dott/1 -> MATLAB Function/7(s_dot)
  U_ss/1 -> MATLAB Function/9(U_ss)
  eta_dss/1 -> MATLAB Function/8(eta_dss)
  MATLAB Function/1(alpha_1dott) -> alpha_1dott/1
  z_1/1 -> MATLAB Function/10(z_1)

== system ModelPlant_DP_v3/Subsystem1/PathParameterization/PathGenerization_Ellips/Path parametization /Subsystem ==
  Elipscenter_radi : Inport
  s : Inport  Port=2
  U_ref : Inport  Port=3
  MATLAB Function : MATLAB Function  TreatAsAtomicUnit=on
  Reshape1 : Reshape  OutputDimensionality=Customize  OutputDimensions=[2,1]
  Reshape2 : Reshape  OutputDimensionality=Customize  OutputDimensions=[3,1]
  Reshape3 : Reshape  OutputDimensionality=Customize  OutputDimensions=[3,1]
  Scope : Scope
      settings: YMin=0.05  YMax=0.4
  P_d : Outport
  Pd_s : Outport  Port=2
  eta_ds : Outport  Port=3
  eta_dss : Outport  Port=4
  U_ss : Outport  Port=5
  wires:
  MATLAB Function/1(pd) -> P_d/1
  Reshape1/1 -> Pd_s/1
  Elipscenter_radi/1 -> MATLAB Function/1(Elipscenter_radi)
  s/1 -> Scope/1, MATLAB Function/2(s)
  Reshape2/1 -> eta_ds/1
  MATLAB Function/2(pd_s) -> Reshape1/1
  MATLAB Function/3(eta_ds) -> Reshape2/1
  MATLAB Function/4(eta_dss) -> Reshape3/1
  Reshape3/1 -> eta_dss/1
  U_ref/1 -> MATLAB Function/3(U_ref)
  MATLAB Function/5(U_ss) -> U_ss/1

== system ModelPlant_DP_v3/Subsystem1/PathParameterization/PathGenerization_Straight/Path parametization /Eta_ds ==
  s : Inport
  p_ds : Inport  Port=2
  Constant : Constant  Value=0
  Constant1 : Constant  Value=0
  Demux : Demux  Outputs=2
  MATLAB Function : MATLAB Function  TreatAsAtomicUnit=on
  MATLAB Function1 : MATLAB Function  Commented=on  TreatAsAtomicUnit=on
  Memory s : Memory  Commented=on
  Memory x_d : Memory  Commented=on
  Memory y_d : Memory  Commented=on
  Mux : Mux  Inputs=2
  eta_ds : Outport
  wires:
  MATLAB Function1/2(y_dd) -> Memory y_d/1
  Demux/1 -> MATLAB Function/1(x_d), MATLAB Function1/1(x_d)
  Mux/1 -> eta_ds/1
  Demux/2 -> MATLAB Function1/2(y_d), MATLAB Function/2(y_d)
  s/1 -> MATLAB Function1/3(s)
  p_ds/1 -> Mux/1, Demux/1
  MATLAB Function1/1(x_dd) -> Memory x_d/1
  Memory y_d/1 -> MATLAB Function1/5(y_dPrev)
  Memory x_d/1 -> MATLAB Function1/4(x_dPrev)
  Memory s/1 -> MATLAB Function1/6(s_Prev)
  MATLAB Function1/3(s1) -> Memory s/1
  MATLAB Function/1(eta_ds_yaw) -> Mux/2
  Constant/1 -> MATLAB Function/3(x_dd)
  Constant1/1 -> MATLAB Function/4(y_dd)

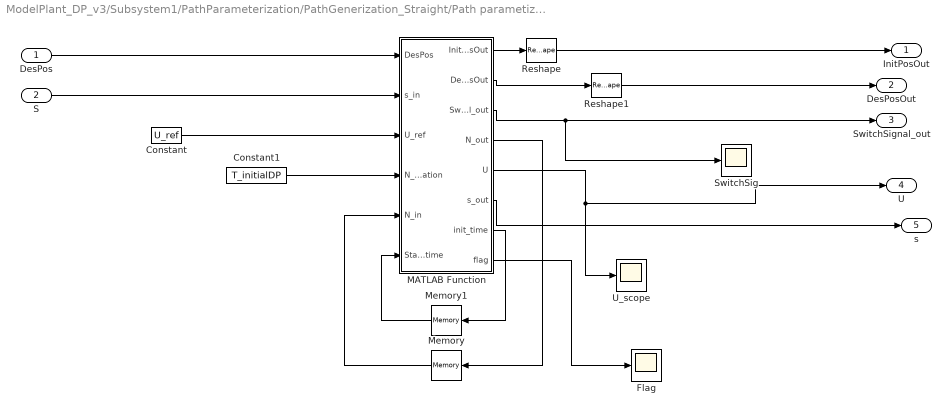
== system ModelPlant_DP_v3/Subsystem1/PathParameterization/PathGenerization_Straight/Path parametization /Subsystem ==
  DesPos : Inport
  S : Inport  Port=2
  Constant : Constant  Value=U_ref
  Constant1 : Constant  Value=T_initialDP
  Flag : Scope
      settings: YMin=0  YMax=50  SaveName=ScopeData17
  MATLAB Function : MATLAB Function  TreatAsAtomicUnit=on
  Memory : Memory  X0=1
  Memory1 : Memory  X0=[0,0]
  Reshape : Reshape  OutputDimensionality=Customize  OutputDimensions=[2,1]
  Reshape1 : Reshape  OutputDimensionality=Customize  OutputDimensions=[2,1]
  SwitchSig : Scope
      settings: SaveName=ScopeData18
  "U_scope " : Scope
      settings: YMin=-1  YMax=1  SaveName=ScopeData16
  InitPosOut : Outport
  DesPosOut : Outport  Port=2
  SwitchSignal_out : Outport  Port=3
  U : Outport  Port=4
  s : Outport  Port=5
  wires:
  MATLAB Function/1(InitPosOut) -> Reshape/1
  MATLAB Function/2(DesPosOut) -> Reshape1/1
  DesPos/1 -> MATLAB Function/1(DesPos)
  S/1 -> MATLAB Function/2(s_in)
  Memory/1 -> MATLAB Function/5(N_in)
  MATLAB Function/4(N_out) -> Memory/1
  MATLAB Function/3(SwitchSignal_out) -> SwitchSignal_out/1, SwitchSig/1
  Reshape/1 -> InitPosOut/1
  Reshape1/1 -> DesPosOut/1
  Constant/1 -> MATLAB Function/3(U_ref)
  MATLAB Function/6(s_out) -> s/1
  MATLAB Function/5(U) -> U/1, "U_scope "/1
  Constant1/1 -> MATLAB Function/4(N_iteration)
  MATLAB Function/7(init_time) -> Memory1/1
  Memory1/1 -> MATLAB Function/6(Start_time)
  MATLAB Function/8(flag) -> Flag/1

== matlab function ModelPlant_DP_v3/safety zone /KillSwitch ==
  data: tau output; eta input; Kill_signal output; lim_2 input; tau_inn input; kill_inn input
function [tau,Kill_signal] = fcn(eta,lim_2,tau_inn,kill_inn)

if kill_inn==1;
    Kill_signal=1;
    %disp('Flag 3.0 KILL - previous kill');
else
    if eta(1)>=lim_2(1)
        Kill_signal=1;
        X=1;
        %disp('Flag 3.1 KILL - large x');
    elseif eta(1)<=lim_2(2)
        Kill_signal=1;
        X=1;
        %disp('Flag 3.2 KILL - small x');
    else
        Kill_signal=0;
        X=0;
    end %IF
    if eta(2)>=lim_2(3)
        Kill_signal=1;
        %disp('Flag 3.3 KILL - large y');
    elseif eta(2)<=lim_2(4)
        Kill_signal=1;
        %disp('Flag 3.4 KILL - small y');
    else
        if X==1
            Kill_signal=1;
        else
            Kill_signal=0; 
        end
        
    end %IF
end% IF

if Kill_signal==1
    tau=[0;0;0];
else
    tau=tau_inn;    
end %IF


end %Function

== matlab function ModelPlant_DP_v3/Subsystem1/Controller1/Control parameterization/BacksteppingParameterization /V_1s/MATLAB Function ==
  data: z_1 input; z_1T output
function z_1T = fcn(z_1)

z_1T=z_1';
end

== matlab function ModelPlant_DP_v3/Subsystem1/Controller1/Control parameterization/BacksteppingParameterization /V_1s/MATLAB Function1 ==
  data: R input; R_T output
function R_T = fcn(R)

R_T=transpose(R);

end

== matlab function ModelPlant_DP_v3/Subsystem1/Controller1/Controller/Controller/MATLAB Function ==
  data: u input; D output; v input; r input
function D = fcn(u,v,r)
%% Damping coefficients
% Comments at the end of the lines indicate the old values used.
X_u		= -0.6555;		X_v		= 0;
X_uu 	= 0.3545;		X_vv	= -2.443;
X_uuu 	= -3.787;		X_vvv	= 0;

Y_v		= -1.33; 			Y_r		= -7.250; % Y_r
Y_vv	= -2.776;			Y_rr	= -3.450; % Y_rr
Y_vvv	= -64.91;			Y_rrr	= 0;
						
Y_rv	= -0.805;			Y_vr	= -0.845; % Y_rv, Y_vr

N_v		= 0;				N_r		= -1.900; % N_r
N_vv	= -0.2088;			N_rr	= -0.750; % N_rr
N_vvv	= 0;				N_rrr	= 0;
N_rv	= 0.130;			N_vr	= 0.080; % N_rv, N_vr
d_11 = -X_u - X_uu*u - X_uuu*u^2;
d_22 = -Y_v - Y_vv*v - Y_vvv*v^2 - Y_rv*abs(r);
d_33 = -N_r - N_rr*abs(r) - N_rrr*r^2 - N_vr*abs(v); % using abs(r)

d_12 = -X_v - X_vv*v - X_vvv*v^2;
d_23 = -Y_r - Y_rr*abs(r) - Y_rrr*r^2 - Y_vr*abs(v);
d_32 = -N_v - N_vv*v - N_vvv*v^2 - N_rv*abs(r);

D    = [d_11 0    0
        0    d_22 d_23
        0    d_32 d_33];
end

== matlab function ModelPlant_DP_v3/safety zone /MATLAB Function ==
  data: kill_signalInn input; kill_signal output; Comand input
function kill_signal = fcn(kill_signalInn,Comand)

if Comand==1
    kill_signal=0;
else
    kill_signal=kill_signalInn;
end

end

== matlab function ModelPlant_DP_v3/Subsystem1/Controller1/Controller/Controller/MATLAB Function1 ==
  data: m input; M output
function M = fcn(m)
%% MATRICES

   I_z  =  1.7600;   x_g = 0.0375;       % x_g  =  0.0460; % Table B.1


%% Added mass
X_ud  =     -2.0;											% Table B.1
					Y_vd =     -1.0;	N_vd =    -0.0;		% Table B.1 guestimate
					Y_rd =      -0.0;	N_rd =    -1.0;		% Table B.1

%% Total mass matrix
m_11 = m-X_ud;
m_22 = m-Y_vd;
m_23 = m*x_g-Y_rd;
m_32 = m*x_g-N_vd;
m_33 = I_z-N_rd;

M    = [m_11 0    0
        0    m_22 m_23
        0    m_32 m_33];
end

== matlab function ModelPlant_DP_v3/Subsystem1/Controller1/Controller/Controller/alpha_1dott/MATLAB Function ==
  data: K_1 input; alpha_1dott output; nu input; r input; eta_ds input; R_T input; U_s input; s_dot input; eta_dss input; U_ss input; z_1 input
function alpha_1dott = fcn(K_1,nu,r,eta_ds,R_T,U_s,s_dot,eta_dss,U_ss,z_1)
%% term 1
S_T=[0 r 0;-r 0 0;0 0 0];

term1=S_T*R_T*eta_ds*U_s;
%% term 2

term2=K_1*(-S_T*z_1-nu);
%% term 3

term3=K_1*R_T*eta_ds*s_dot;
%% term 4

term4=R_T*eta_dss*s_dot*U_s;
%% term 5 

term5=R_T*eta_ds*U_ss*s_dot;
%% summary

alpha_1dott=term1+term2+term3+term4+term5;
end

== matlab function ModelPlant_DP_v3/safety zone /Safety Act ==
  data: joyStick input; safetySig_1 input; safetySig_2 input; safetySig_3 input; safetySig_4 input; thrust_out output; vel input; switch_sig output; K input
function [thrust_out,switch_sig] = fcn(joyStick,safetySig_1,safetySig_2,safetySig_3,safetySig_4,vel,K)

switch_sig=0;
thrust_out=zeros(3,1);
%K=[1;1];    

    if safetySig_1 == 0 && safetySig_2 == 0 && safetySig_3 == 0 && safetySig_4 == 0   %Check to see if intervention is requiered
        
    switch_sig = 0; %Intervention is NOT requiered
    ThrustX=joyStick(1);
    ThrustY=joyStick(2);
       %disp('Flag 0.0 All OK - No safety sig');
    else
    switch_sig=1;   %Intervention IS requiered
    
        if  safetySig_1==1 || safetySig_2==1 %Problem in X dir
            %disp('Flag 1.0 Problem in x');
            if joyStick(1)==0 %Check if inputforce fore is zero or correct, (but the velocity might not be)
               %Perhaps a proprtional gain depending on the velocity?
               if vel(1)<0 && safetySig_2==1
                   ThrustX=K(1)*-vel(1);
                   %disp('Flag 1.1 (x - tau=0 - Negative vel + to low x pos -> thrust =-vel*K_1)');
               elseif vel(1)> 0 && safetySig_1==1
                   ThrustX=K(1)*-vel(1);
                   %disp('Flag 1.2 (x - tau=0 - Positive vel + to high x pos -> thrust =-vel*K_1)');
               else
                   ThrustX=K(1)*vel(1);
                   %disp('Flag 1.3 (x - tau=0 - Positive vel + to low x pos / Negative vel + to highx pos -> keep current trust)');
               end
                %thrust_out=[ThrustX;joyStick(2);joyStick(3)];
                
            elseif joyStick(1) >0 && safetySig_2==1     %X cord to small, but thrust right way
                ThrustX=joyStick(1);
                %thrust_out=[joyStick(1);joyStick(2);joyStick(3)];
                %disp('Flag 1.4 (x - Positive thrust + to low x post -> keep current trust)');
            elseif joyStick(1) <0 && safetySig_1==1     %X cord to large, but thrust right way
                ThrustX=joyStick(1);
                %thrust_out=[joyStick(1);joyStick(2);joyStick(3)];
                %disp('Flag 1.5 (x - Negative thrust + to high x post -> Keep current trust)');
            else
                ThrustX=-joyStick(1);
                %thrust_out=[-joyStick(1);joyStick(2);joyStick(3)];
                %disp('Flag 1.6 (x - Negative thrust + to low x post / Positive thrust + to high x post -> reverse trust)');
            end %If
        else
            ThrustX=joyStick(1);
        end %IF  
        
        if  safetySig_3==1 || safetySig_4==1 %Problem in X dir%Problem in Y dir
            %disp('Flag 2.0 Problem in y');
            if joyStick(2)==0 %Check if inputforce fore is zero or correct
                %Perhaps a proprtional gain depending on the velocity?  
                if vel(2)>0 && safetySig_3==1
                    ThrustY=K(2)*-vel(2);
                    %disp('Flag 2.1 (y - tau=0 - Negative vel + to low y pos -> thrust =-vel*K_2)');
                elseif vel(2)< 0 && safetySig_4==1
                    ThrustY=K(2)*-vel(2);
                    %disp('Flag 2.2 (y - tau=0 - Positive vel + to high y pos -> thrust =-vel*K_2)');
                else
                    ThrustY=K(2)*vel(2);
                    %disp('Flag 2.3 (y - tau=0 - Positive vel + to low y pos / Negative vel + to high y pos -> keep current trust)');
                end %IF
                %thrust_out=[joyStick(1);ThrustY;joyStick(3)];
                  
            elseif joyStick(2) >0 && safetySig_4==1     %Y cord to small
                ThrustY=joyStick(2);
                %thrust_out=[joyStick(1);joyStick(2);joyStick(3)];
                %disp('Flag 2.4 (y - Positive thrust + to low y post -> keep current trust)');
                
            elseif joyStick(2) <0 && safetySig_3==1     %Y cord to large
                ThrustY=joyStick(2);
                %thrust_out=[joyStick(1);joyStick(2);joyStick(3)];
                %disp('Flag 2.5 (y - Negative thrust + to high y post -> Keep current trust)');
                
            else
                ThrustY=-joyStick(2);
            %thrust_out=[joyStick(1);-joyStick(2);joyStick(3)];
            %disp('Flag 2.6 (y - Negative thrust + to low y post / Positive thrust + to high y post -> reverse trust)');
            
            end %IF
        else
            ThrustY=joyStick(2);
        end %IF
        
    end %IF
        thrust_out=[ThrustX;ThrustY;joyStick(3)];
end %Function

== matlab function ModelPlant_DP_v3/safety zone /safety check ==
  data: eta input; safety_sig_1 output; safety_sig_2 output; safety_sig_3 output; safety_sig_4 output; lim input
function [safety_sig_1,safety_sig_2,safety_sig_3,safety_sig_4]= fcn(eta,lim)


%safety_sig=[0;0;0;0];%orginal safety signal
%lim=[40.00;0;6.45;0];%space limitation [x_max;x_min;y_max;y_min]
if eta(1)>=lim(1)
    safety_sig_1 = 1;
    safety_sig_2= 0;
elseif eta(1)<=lim(2)
    safety_sig_2 = 1;
    safety_sig_1=0;
else
    safety_sig_1 = 0;
    safety_sig_2 = 0;
end
if eta(2)>lim(3)
    safety_sig_3 = 1;
    safety_sig_4 = 0;
elseif eta(2)<lim(4)
    safety_sig_4 = 1;
    safety_sig_3 = 0;

else
    safety_sig_3 = 0;
    safety_sig_4 = 0;
end
% safety_sig_1=safety_sig(1);
% safety_sig_2=safety_sig(2);
%safety_sig_3=safety_sig(3);
%safety_sig_4=safety_sig(4);

end

== matlab function ModelPlant_DP_v3/physics_model/kinematics ==
  data: nu input; eta_dot output; eta input
function eta_dot = CSE1_eta_dot(nu,eta)

psi = eta(3);

J = [cos(psi) -sin(psi) 0
     sin(psi) cos(psi)  0
     0        0         1];

eta_dot = J*nu;
end

== matlab function ModelPlant_DP_v3/physics_model/kinetics ==
  data: tau input; nu_dot output; nu input
function nu_dot = CSE1_nu_dot_corr(tau,nu)

u   = nu(1);
v   = nu(2);
r   = nu(3);

tau = [tau(1);tau(2);tau(3)];
%% MATRICES

m    = 14.79;   I_z  =  1.7600;   x_g = 0.0375;       % x_g  =  0.0460; % Table B.1


%% Added mass
X_ud  =     -2.0;											% Table B.1
Y_vd =     -10.0;	
N_vd =    -0.0;                                             % Table B.1 guestimate
Y_rd =      -0.0;	
N_rd =    -1.0;                                             % Table B.1

%% Total mass matrix
m_11 = m-X_ud;
m_22 = m-Y_vd;
m_23 = m*x_g-Y_rd;
m_32 = m*x_g-N_vd;
m_33 = I_z-N_rd;

M    = [m_11 0    0
        0    m_22 m_23
        0    m_32 m_33];
	
%% Damping coefficients
% Comments at the end of the lines indicate the old values used.
X_u		= -0.6555;		X_v		= 0;
X_uu 	= 0.3545;		X_vv	= -2.443;
X_uuu 	= -3.787;		X_vvv	= 0;

Y_v		= -1.33; 			Y_r		= -7.250; % Y_r
Y_vv	= -2.776;			Y_rr	= -3.450; % Y_rr
Y_vvv	= -64.91;			Y_rrr	= 0;
						
Y_rv	= -0.805;			Y_vr	= -0.845; % Y_rv, Y_vr

N_v		= 0;				N_r		= -1.900; % N_r
N_vv	= -0.2088;			N_rr	= -0.750; % N_rr
N_vvv	= 0;				N_rrr	= 0;
N_rv	= 0.130;			N_vr	= 0.080; % N_rv, N_vr

%% Correolis matrix

%from ItsLearning
% c_13 = -(m-Y_vd)*v-(m*x_g-Y_rd)*r;
% c_23 = (m-X_ud)*u;
% C    = [0     0     c_13
%         0     0     c_23
%         -c_13 -c_23 0   ];

%From Handbook of Marine Craft Hydr 1st ed pp.120
a1 = X_ud*u;
a2 = Y_vd*v-m*x_g*r;
C    = [0     0     a2
        0     0    -a1
       -a2    a1    0   ];

%% Assembly of the damping matrix
d_11 = -X_u - X_uu*u - X_uuu*u^2;
d_22 = -Y_v - Y_vv*v - Y_vvv*v^2 - Y_rv*abs(r);
d_33 = -N_r - N_rr*abs(r) - N_rrr*r^2 - N_vr*abs(v); % using abs(r)

d_12 = -X_v - X_vv*v - X_vvv*v^2;
d_23 = -Y_r - Y_rr*abs(r) - Y_rrr*r^2 - Y_vr*abs(v);
d_32 = -N_v - N_vv*v - N_vvv*v^2 - N_rv*abs(r);

%From ItsLearning
% D    = [d_11 d_12 0
%         0    d_22 d_23
%         0    d_32 d_33];

%From Feb. 2017 lab manual. Agrees with Handbook of Marine Craft Hydro
D    = [d_11 0    0
        0    d_22 d_23
        0    d_32 d_33];



%% CALCULATION

%nu_dot = M\(tau-(C+D)*nu);
nu_dot = M\(tau-(D)*nu);

== matlab function ModelPlant_DP_v3/safety zone /MATLAB Function1 ==
  data: R input; R_T output
function R_T = fcn(R)
R_T=transpose(R);
end

== matlab function ModelPlant_DP_v3/Subsystem1/Controller1/Control parameterization/BacksteppingParameterization /V_1s/Rotation Matrix ==
  data: yaw input; R output
function R = fcn(yaw)

R=[cos(yaw) -sin(yaw) 0;
    sin(yaw) cos(yaw) 0;
    0 0 1];

end

== matlab function ModelPlant_DP_v3/Subsystem1/Controller1/Control parameterization/BacksteppingParameterization /Z_1/R Transposed ==
  data: R input; R_T output
function R_T = fcn(R)

R_T=transpose(R);

end

== matlab function ModelPlant_DP_v3/Subsystem1/Controller1/Control parameterization/BacksteppingParameterization /Z_1/Rotation Matrix ==
  data: yaw input; R output
function R = fcn(yaw)

R=[cos(yaw) -sin(yaw) 0;
    sin(yaw) cos(yaw) 0;
    0 0 1];

end

== matlab function ModelPlant_DP_v3/Subsystem1/PathParameterization/PathGenerization_Ellips/Check_s/CheckS&getU ==
  data: s_inn input; s_out output; U output; U_ref input; Switch output
function [s_out,U,Switch]= fcn(s_inn,U_ref)

if s_inn>=1
    s_out=0;
    Switch=0;
else
    s_out=s_inn;
    Switch=1;
end

U=U_ref/2;%U scaled again for the ellipsoidal case

end

== matlab function ModelPlant_DP_v3/Subsystem1/PathParameterization/PathGenerization_Straight/Path parametization /Eta_ds/MATLAB Function ==
  data: x_d input; eta_ds_yaw output; y_d input; x_dd input; y_dd input
function eta_ds_yaw = fcn(x_d,y_d,x_dd,y_dd)

eta_ds_yaw=(x_d*y_dd-y_d*x_dd)/(y_d^2+x_d^2);

end

== matlab function ModelPlant_DP_v3/Subsystem1/PathParameterization/PathGenerization_Straight/Path parametization /Eta_ds/MATLAB Function1 ==
  data: x_d input; x_dd output; y_d input; s input; y_dd output; x_dPrev input; y_dPrev input; s_Prev input; s1 output
function [x_dd,y_dd,s1]= fcn(x_d,y_d,s,x_dPrev,y_dPrev,s_Prev)

Delta_x=x_d-x_dPrev;
Delta_y=y_d-y_dPrev;
Delta_s=s-s_Prev;


x_dd=Delta_x/Delta_s;
y_dd=Delta_y/Delta_s;

s1=s;

end

== matlab function ModelPlant_DP_v3/Subsystem1/PathParameterization/PathGenerization_Ellips/Path parametization /Subsystem/MATLAB Function ==
  data: Elipscenter_radi input; pd output; s input; pd_s output; eta_ds output; eta_dss output; U_ref input; U_ss output
function [pd,pd_s,eta_ds,eta_dss,U_ss] = fcn(Elipscenter_radi,s,U_ref)
pd=zeros(2,1);
pd_s=pd;
eta_ds=zeros(3,1);
eta_dss=zeros(3,1);

pd(1)=Elipscenter_radi(1,1)+cos(2*pi*s)*Elipscenter_radi(1,2);
pd(2)=Elipscenter_radi(2,1)+sin(2*pi*s)*Elipscenter_radi(2,2);

pd_s(1)=-2*pi*Elipscenter_radi(1,2)*sin(2*pi*s);
pd_s(2)=2*pi*Elipscenter_radi(2,2)*cos(2*pi*s);

eta_ds(1)=pd_s(1);
eta_ds(2)=pd_s(2);
x_dss=-4*pi^2*Elipscenter_radi(1,2)*cos(2*pi*s);
y_dss=-4*pi^2*Elipscenter_radi(2,2)*sin(2*pi*s);
x_ds=pd_s(1);
y_ds=pd_s(2);
eta_ds(3)=(x_ds*y_dss-x_dss*y_ds)/(x_ds^2+y_ds^2);
eta_dss(1)=x_dss;
eta_dss(2)=y_dss;

x_dsss=8*pi^3*Elipscenter_radi(1,2)*sin(2*pi*s);
y_dsss=-8*pi^3*Elipscenter_radi(2,2)*cos(2*pi*s);
term1=(x_ds*y_dsss-y_ds*x_dsss)/(x_ds^2+y_ds^2);
term2=-((x_ds*y_dss-y_ds*x_dss)*(2*x_ds*x_dss+2*y_ds*y_dss))/(x_ds^2+y_ds^2)^2;
eta_dss(3)=term1+term2;
U_ss=U_ref*(-x_ds*x_dss-y_ds*y_dss)/((x_ds^2+y_ds^2)^(1.5));
end

== matlab function ModelPlant_DP_v3/Subsystem1/PathParameterization/PathGenerization_Ellips/parameter generator/MATLAB Function1 ==
  data: SwitchSignal_In input; SwitchSignal_Out output
function SwitchSignal_Out = fcn(SwitchSignal_In)

if SwitchSignal_In==0
    SwitchSignal_Out=1;
else
    SwitchSignal_Out=0;
end
    
end
